simulink library "DaVinci_LibJ_Trajectory"  (R2023a)
settings: Solver=VariableStepAuto  StartTime=0.0  StopTime=10.0  RelTol=1e-3
settings Model: Creator=afons  LastModifiedBy=afons

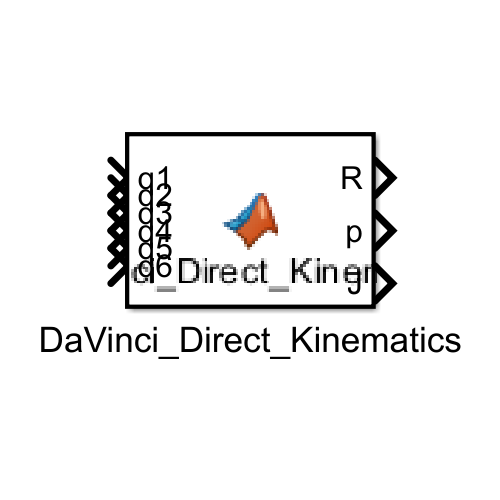
[thumbnail: Simulink's stored preview of the top-level diagram]
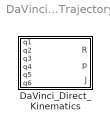
== system DaVinci_LibJ_Trajectory ==
  DaVinci_Direct_Kinematics : MATLAB Function  TreatAsAtomicUnit=on

== matlab function DaVinci_LibJ_Trajectory/DaVinci_Direct_Kinematics ==
  data: q1 input; R output; q2 input; q3 input; q4 input; q5 input; q6 input; p output; J output
function [R,p,J] = DaVinci_Direct_Kinematics(q1,q2,q3,q4,q5,q6)
%#codegen

%    This function was generated by the Symbolic Math Toolbox version 9.3.
%    26-May-2023 11:46:51

% q1 = complex(q1);  % if required to enforce complex operations
% q2 = complex(q2);  % if required to enforce complex operations
% q3 = complex(q3);  % if required to enforce complex operations
% q4 = complex(q4);  % if required to enforce complex operations
% q5 = complex(q5);  % if required to enforce complex operations
% q6 = complex(q6);  % if required to enforce complex operations
t2 = cos(q1);
t3 = cos(q2);
t4 = cos(q4);
t5 = cos(q5);
t6 = cos(q6);
t7 = sin(q1);
t8 = sin(q2);
t9 = sin(q4);
t10 = sin(q5);
t11 = sin(q6);
t12 = t6.*2.0;
t13 = t2.*t3;
t14 = t3.*t7;
t15 = t5.*t8;
t16 = t8.*t10;
t23 = q3.*t8.*1.0e+2;
t24 = t2.*t4.*t5;
t26 = t4.*t5.*t7;
t27 = t3.*t5.*t9;
t29 = t3.*t9.*t10;
t31 = t3.*t4.*t11.*2.0;
t39 = (t7.*t9.*t11)./5.0e+1;
t43 = (t2.*t9.*t11)./5.0e+1;
t47 = (t2.*t4.*t10)./1.0e+2;
t48 = (t4.*t7.*t10)./1.0e+2;
t51 = (t2.*t4.*t6.*t10)./5.0e+1;
t52 = (t2.*t4.*t8.*t11)./5.0e+1;
t53 = (t4.*t6.*t7.*t10)./5.0e+1;
t55 = (t4.*t7.*t8.*t11)./5.0e+1;
t17 = q3.*t13;
t18 = q3.*t14;
t19 = t12+1.0;
t20 = -t13;
t21 = -t14;
t22 = -t16;
t25 = t10.*t13;
t28 = t10.*t14;
t32 = t12.*t15;
t33 = t2.*t9.*t15;
t34 = t7.*t9.*t15;
t35 = -t26;
t36 = -t27;
t37 = -t29;
t41 = t6.*t29.*-2.0;
t44 = -t39;
t45 = (t5.*t13)./1.0e+2;
t46 = (t5.*t14)./1.0e+2;
t49 = (t5.*t6.*t13)./5.0e+1;
t50 = (t5.*t6.*t14)./5.0e+1;
t56 = -t48;
t58 = -t53;
t59 = (t2.*t9.*t16)./1.0e+2;
t60 = (t7.*t9.*t16)./1.0e+2;
t61 = (t2.*t6.*t9.*t16)./5.0e+1;
t62 = (t6.*t7.*t9.*t16)./5.0e+1;
t30 = -t17;
t40 = -t33;
t42 = -t34;
t54 = -t45;
t57 = -t49;
t63 = -t59;
t64 = -t61;
t65 = t22+t36;
t68 = t15+t23+t31+t32+t37+t41;
t66 = t24+t28+t42;
t67 = t25+t35+t40;
R = reshape([-t7.*t9.*t11+t5.*t6.*t20+t2.*t4.*t8.*t11-t4.*t6.*t7.*t10+t2.*t6.*t9.*t22,t2.*t9.*t11+t5.*t6.*t21+t2.*t4.*t6.*t10+t4.*t7.*t8.*t11+t6.*t7.*t9.*t22,t6.*t15+t6.*t37+t3.*t4.*t11,-t6.*t7.*t9+t5.*t11.*t13+t2.*t4.*t6.*t8+t4.*t7.*t10.*t11+t2.*t9.*t11.*t16,t2.*t6.*t9+t5.*t11.*t14+t4.*t6.*t7.*t8-t2.*t4.*t10.*t11+t7.*t9.*t11.*t16,-t11.*t15+t11.*t29+t3.*t4.*t6,t67,t66,t65],[3,3]);
if nargout > 1
    t69 = t30+t44+t52+t54+t56+t57+t58+t63+t64;
    p = [t69;-t18+t43-t46+t47-t50+t51+t55-t60-t62;t15./1.0e+2-t29./1.0e+2+q3.*t8+(t6.*t15)./5.0e+1-(t6.*t29)./5.0e+1+(t3.*t4.*t11)./5.0e+1];
end
if nargout > 2
    mt1 = [t18-t43+t46-t47+t50-t51-t55+t60+t62,t69,0.0,0.0,0.0,1.0,(t2.*t68)./1.0e+2,(t7.*t68)./1.0e+2,q3.*t3+(t3.*t5)./1.0e+2+(t9.*t16)./1.0e+2+(t3.*t5.*t6)./5.0e+1-(t4.*t8.*t11)./5.0e+1+(t6.*t9.*t16)./5.0e+1,-t7,t2,0.0,t20,t21,t8,0.0,0.0,0.0,t2.*t4.*t16.*(-1.0./1.0e+2)-(t4.*t7.*t11)./5.0e+1+(t7.*t9.*t10)./1.0e+2-(t2.*t4.*t6.*t16)./5.0e+1-(t2.*t8.*t9.*t11)./5.0e+1+(t6.*t7.*t9.*t10)./5.0e+1];
    mt2 = [(t2.*t4.*t11)./5.0e+1-(t2.*t9.*t10)./1.0e+2-(t4.*t7.*t16)./1.0e+2-(t2.*t6.*t9.*t10)./5.0e+1-(t4.*t6.*t7.*t16)./5.0e+1-(t7.*t8.*t9.*t11)./5.0e+1,t3.*(t4.*t10+t9.*t11.*2.0+t4.*t10.*t12).*(-1.0./1.0e+2),t20,t21,t8,t19.*(t26+t33+t10.*t20).*(-1.0./1.0e+2),(t19.*t66)./1.0e+2,t19.*(t16+t27).*(-1.0./1.0e+2),t7.*t9-t2.*t4.*t8,-t2.*t9-t4.*t7.*t8,-t3.*t4,t16.*t43-(t6.*t7.*t9)./5.0e+1+(t5.*t11.*t13)./5.0e+1+(t2.*t4.*t6.*t8)./5.0e+1+(t4.*t7.*t10.*t11)./5.0e+1];
    mt3 = [t16.*t39+(t2.*t6.*t9)./5.0e+1+(t5.*t11.*t14)./5.0e+1+(t4.*t6.*t7.*t8)./5.0e+1-(t2.*t4.*t10.*t11)./5.0e+1,t11.*t15.*(-1.0./5.0e+1)+(t11.*t29)./5.0e+1+(t3.*t4.*t6)./5.0e+1,t67,t66,t65];
    J = reshape([mt1,mt2,mt3],6,6);
end
end
